simulink model "rx2"  (R2022b)
settings: Solver=FixedStepDiscrete  StartTime=0.0  StopTime=3.3E6  FixedStep=1  RelTol=1e-3  EnableMultiTasking=on
model workspace (MAT data in the model file):
  mwTaskManagerKernelLatency = 0
undefined symbols (not defined in the file or in its folder): Add, jsin, magnitude, rom_pilot_conj_tt, Shift
libraries: hdlsllib x3231, whdlutilities x525, simulink x260, whdlmod x112, whdledac x26, dsphdlmathfun2 x24, commchan3 x1
(part 19 of 59)

== system rx2/process divide/transport_block8/Subsystem4/ctrl_gen ==
  data_in : Inport
  valid_in : Inport  Port=2
  Delay : Delay  DelayLength=1  InitialCondition=0
  Delay1 : Delay  DelayLength=1  InitialCondition=0
  Delay2 : Delay  DelayLength=1  InitialCondition=0
  Detect Fall Nonpositive : hdlsllib/Logic and Bit Operations/Detect Fall Nonpositive  vinit=0  OutDataTypeStr=boolean
  Detect Rise Positive : hdlsllib/Logic and Bit Operations/Detect Rise Positive  vinit=0  OutDataTypeStr=boolean
  Sample Control Bus Creator : whdlutilities/Sample Control Bus Creator
  data_out : Outport
  ctrl_out : Outport  Port=2
  wires:
  Detect Fall Nonpositive/1 -> Sample Control Bus Creator/2
  valid_in/1 -> Delay/1, Detect Fall Nonpositive/1, Delay1/1
  Sample Control Bus Creator/1 -> ctrl_out/1
  Delay/1 -> Sample Control Bus Creator/3
  Delay1/1 -> Detect Rise Positive/1
  data_in/1 -> Delay2/1
  Delay2/1 -> data_out/1
  Detect Rise Positive/1 -> Sample Control Bus Creator/1

== system rx2/process divide/transport_block8/Subsystem5/ctrl_gen ==
  data_in : Inport
  valid_in : Inport  Port=2
  Delay : Delay  DelayLength=1  InitialCondition=0
  Delay1 : Delay  DelayLength=1  InitialCondition=0
  Delay2 : Delay  DelayLength=1  InitialCondition=0
  Detect Fall Nonpositive : hdlsllib/Logic and Bit Operations/Detect Fall Nonpositive  vinit=0  OutDataTypeStr=boolean
  Detect Rise Positive : hdlsllib/Logic and Bit Operations/Detect Rise Positive  vinit=0  OutDataTypeStr=boolean
  Sample Control Bus Creator : whdlutilities/Sample Control Bus Creator
  data_out : Outport
  ctrl_out : Outport  Port=2
  wires:
  Detect Fall Nonpositive/1 -> Sample Control Bus Creator/2
  valid_in/1 -> Delay/1, Detect Fall Nonpositive/1, Delay1/1
  Sample Control Bus Creator/1 -> ctrl_out/1
  Delay/1 -> Sample Control Bus Creator/3
  Delay1/1 -> Detect Rise Positive/1
  data_in/1 -> Delay2/1
  Delay2/1 -> data_out/1
  Detect Rise Positive/1 -> Sample Control Bus Creator/1

== system rx2/process divide/transport_block8/Subsystem6/ctrl_gen ==
  data_in : Inport
  valid_in : Inport  Port=2
  Delay : Delay  DelayLength=1  InitialCondition=0
  Delay1 : Delay  DelayLength=1  InitialCondition=0
  Delay2 : Delay  DelayLength=1  InitialCondition=0
  Detect Fall Nonpositive : hdlsllib/Logic and Bit Operations/Detect Fall Nonpositive  vinit=0  OutDataTypeStr=boolean
  Detect Rise Positive : hdlsllib/Logic and Bit Operations/Detect Rise Positive  vinit=0  OutDataTypeStr=boolean
  Sample Control Bus Creator : whdlutilities/Sample Control Bus Creator
  data_out : Outport
  ctrl_out : Outport  Port=2
  wires:
  Detect Fall Nonpositive/1 -> Sample Control Bus Creator/2
  valid_in/1 -> Delay/1, Detect Fall Nonpositive/1, Delay1/1
  Sample Control Bus Creator/1 -> ctrl_out/1
  Delay/1 -> Sample Control Bus Creator/3
  Delay1/1 -> Detect Rise Positive/1
  data_in/1 -> Delay2/1
  Delay2/1 -> data_out/1
  Detect Rise Positive/1 -> Sample Control Bus Creator/1

== system rx2/process divide/transport_block8/Subsystem7/ctrl_gen ==
  data_in : Inport
  valid_in : Inport  Port=2
  Delay : Delay  DelayLength=1  InitialCondition=0
  Delay1 : Delay  DelayLength=1  InitialCondition=0
  Delay2 : Delay  DelayLength=1  InitialCondition=0
  Detect Fall Nonpositive : hdlsllib/Logic and Bit Operations/Detect Fall Nonpositive  vinit=0  OutDataTypeStr=boolean
  Detect Rise Positive : hdlsllib/Logic and Bit Operations/Detect Rise Positive  vinit=0  OutDataTypeStr=boolean
  Sample Control Bus Creator : whdlutilities/Sample Control Bus Creator
  data_out : Outport
  ctrl_out : Outport  Port=2
  wires:
  Detect Fall Nonpositive/1 -> Sample Control Bus Creator/2
  valid_in/1 -> Delay/1, Detect Fall Nonpositive/1, Delay1/1
  Sample Control Bus Creator/1 -> ctrl_out/1
  Delay/1 -> Sample Control Bus Creator/3
  Delay1/1 -> Detect Rise Positive/1
  data_in/1 -> Delay2/1
  Delay2/1 -> data_out/1
  Detect Rise Positive/1 -> Sample Control Bus Creator/1

== system rx2/process divide/transport_block8/Subsystem8/ctrl_gen ==
  data_in : Inport
  valid_in : Inport  Port=2
  Delay : Delay  DelayLength=1  InitialCondition=0
  Delay1 : Delay  DelayLength=1  InitialCondition=0
  Delay2 : Delay  DelayLength=1  InitialCondition=0
  Detect Fall Nonpositive : hdlsllib/Logic and Bit Operations/Detect Fall Nonpositive  vinit=0  OutDataTypeStr=boolean
  Detect Rise Positive : hdlsllib/Logic and Bit Operations/Detect Rise Positive  vinit=0  OutDataTypeStr=boolean
  Sample Control Bus Creator : whdlutilities/Sample Control Bus Creator
  data_out : Outport
  ctrl_out : Outport  Port=2
  wires:
  Detect Fall Nonpositive/1 -> Sample Control Bus Creator/2
  valid_in/1 -> Delay/1, Detect Fall Nonpositive/1, Delay1/1
  Sample Control Bus Creator/1 -> ctrl_out/1
  Delay/1 -> Sample Control Bus Creator/3
  Delay1/1 -> Detect Rise Positive/1
  data_in/1 -> Delay2/1
  Delay2/1 -> data_out/1
  Detect Rise Positive/1 -> Sample Control Bus Creator/1

== system rx2/process divide/transport_block8/Subsystem9/ctrl_gen ==
  data_in : Inport
  valid_in : Inport  Port=2
  Delay : Delay  DelayLength=1  InitialCondition=0
  Delay1 : Delay  DelayLength=1  InitialCondition=0
  Delay2 : Delay  DelayLength=1  InitialCondition=0
  Detect Fall Nonpositive : hdlsllib/Logic and Bit Operations/Detect Fall Nonpositive  vinit=0  OutDataTypeStr=boolean
  Detect Rise Positive : hdlsllib/Logic and Bit Operations/Detect Rise Positive  vinit=0  OutDataTypeStr=boolean
  Sample Control Bus Creator : whdlutilities/Sample Control Bus Creator
  data_out : Outport
  ctrl_out : Outport  Port=2
  wires:
  Detect Fall Nonpositive/1 -> Sample Control Bus Creator/2
  valid_in/1 -> Delay/1, Detect Fall Nonpositive/1, Delay1/1
  Sample Control Bus Creator/1 -> ctrl_out/1
  Delay/1 -> Sample Control Bus Creator/3
  Delay1/1 -> Detect Rise Positive/1
  data_in/1 -> Delay2/1
  Delay2/1 -> data_out/1
  Detect Rise Positive/1 -> Sample Control Bus Creator/1

== system rx2/process1/OFDM_DEMOD1/OFDM_demod1/ctrl_gen ==
  data_in : Inport
  valid_in : Inport  Port=2
  Data Type Conversion : DataTypeConversion  OutDataTypeStr=fixdt(1,16,12)  SaturateOnIntegerOverflow=off  RndMeth=Floor
  Delay : Delay  DelayLength=1  InitialCondition=0
  Delay1 : Delay  DelayLength=1  InitialCondition=0
  Delay2 : Delay  DelayLength=1  InitialCondition=0
  Detect Fall Nonpositive : hdlsllib/Logic and Bit Operations/Detect Fall Nonpositive  vinit=0  OutDataTypeStr=boolean
  Detect Rise Positive : hdlsllib/Logic and Bit Operations/Detect Rise Positive  vinit=0  OutDataTypeStr=boolean
  Sample Control Bus Creator : whdlutilities/Sample Control Bus Creator
  data_out : Outport  OutDataTypeStr=fixdt(1,16,12)
  ctrl_out : Outport  Port=2
  wires:
  Detect Fall Nonpositive/1 -> Sample Control Bus Creator/2
  valid_in/1 -> Delay/1, Detect Fall Nonpositive/1, Delay1/1
  Sample Control Bus Creator/1 -> ctrl_out/1
  Delay/1 -> Sample Control Bus Creator/3
  Delay1/1 -> Detect Rise Positive/1
  data_in/1 -> Delay2/1
  Delay2/1 -> Data Type Conversion/1
  Detect Rise Positive/1 -> Sample Control Bus Creator/1
  Data Type Conversion/1 -> data_out/1

== system rx2/process1/OFDM_DEMOD1/OFDM_demod2/ctrl_gen ==
  data_in : Inport
  valid_in : Inport  Port=2
  Data Type Conversion : DataTypeConversion  OutDataTypeStr=fixdt(1,16,12)  SaturateOnIntegerOverflow=off  RndMeth=Floor
  Delay : Delay  DelayLength=1  InitialCondition=0
  Delay1 : Delay  DelayLength=1  InitialCondition=0
  Delay2 : Delay  DelayLength=1  InitialCondition=0
  Detect Fall Nonpositive : hdlsllib/Logic and Bit Operations/Detect Fall Nonpositive  vinit=0  OutDataTypeStr=boolean
  Detect Rise Positive : hdlsllib/Logic and Bit Operations/Detect Rise Positive  vinit=0  OutDataTypeStr=boolean
  Sample Control Bus Creator : whdlutilities/Sample Control Bus Creator
  data_out : Outport  OutDataTypeStr=fixdt(1,16,12)
  ctrl_out : Outport  Port=2
  wires:
  Detect Fall Nonpositive/1 -> Sample Control Bus Creator/2
  valid_in/1 -> Delay/1, Detect Fall Nonpositive/1, Delay1/1
  Sample Control Bus Creator/1 -> ctrl_out/1
  Delay/1 -> Sample Control Bus Creator/3
  Delay1/1 -> Detect Rise Positive/1
  data_in/1 -> Delay2/1
  Delay2/1 -> Data Type Conversion/1
  Detect Rise Positive/1 -> Sample Control Bus Creator/1
  Data Type Conversion/1 -> data_out/1

== system rx2/process1/OFDM_DEMOD1/OFDM_demod3/ctrl_gen ==
  data_in : Inport
  valid_in : Inport  Port=2
  Data Type Conversion : DataTypeConversion  OutDataTypeStr=fixdt(1,16,12)  SaturateOnIntegerOverflow=off  RndMeth=Floor
  Delay : Delay  DelayLength=1  InitialCondition=0
  Delay1 : Delay  DelayLength=1  InitialCondition=0
  Delay2 : Delay  DelayLength=1  InitialCondition=0
  Detect Fall Nonpositive : hdlsllib/Logic and Bit Operations/Detect Fall Nonpositive  vinit=0  OutDataTypeStr=boolean
  Detect Rise Positive : hdlsllib/Logic and Bit Operations/Detect Rise Positive  vinit=0  OutDataTypeStr=boolean
  Sample Control Bus Creator : whdlutilities/Sample Control Bus Creator
  data_out : Outport  OutDataTypeStr=fixdt(1,16,12)
  ctrl_out : Outport  Port=2
  wires:
  Detect Fall Nonpositive/1 -> Sample Control Bus Creator/2
  valid_in/1 -> Delay/1, Detect Fall Nonpositive/1, Delay1/1
  Sample Control Bus Creator/1 -> ctrl_out/1
  Delay/1 -> Sample Control Bus Creator/3
  Delay1/1 -> Detect Rise Positive/1
  data_in/1 -> Delay2/1
  Delay2/1 -> Data Type Conversion/1
  Detect Rise Positive/1 -> Sample Control Bus Creator/1
  Data Type Conversion/1 -> data_out/1

== system rx2/process1/OFDM_DEMOD1/OFDM_demod4/ctrl_gen ==
  data_in : Inport
  valid_in : Inport  Port=2
  Data Type Conversion : DataTypeConversion  OutDataTypeStr=fixdt(1,16,12)  SaturateOnIntegerOverflow=off  RndMeth=Floor
  Delay : Delay  DelayLength=1  InitialCondition=0
  Delay1 : Delay  DelayLength=1  InitialCondition=0
  Delay2 : Delay  DelayLength=1  InitialCondition=0
  Detect Fall Nonpositive : hdlsllib/Logic and Bit Operations/Detect Fall Nonpositive  vinit=0  OutDataTypeStr=boolean
  Detect Rise Positive : hdlsllib/Logic and Bit Operations/Detect Rise Positive  vinit=0  OutDataTypeStr=boolean
  Sample Control Bus Creator : whdlutilities/Sample Control Bus Creator
  data_out : Outport  OutDataTypeStr=fixdt(1,16,12)
  ctrl_out : Outport  Port=2
  wires:
  Detect Fall Nonpositive/1 -> Sample Control Bus Creator/2
  valid_in/1 -> Delay/1, Detect Fall Nonpositive/1, Delay1/1
  Sample Control Bus Creator/1 -> ctrl_out/1
  Delay/1 -> Sample Control Bus Creator/3
  Delay1/1 -> Detect Rise Positive/1
  data_in/1 -> Delay2/1
  Delay2/1 -> Data Type Conversion/1
  Detect Rise Positive/1 -> Sample Control Bus Creator/1
  Data Type Conversion/1 -> data_out/1

== system rx2/process1/OFDM_DEMOD1/OFDM_demod5/ctrl_gen ==
  data_in : Inport
  valid_in : Inport  Port=2
  Data Type Conversion : DataTypeConversion  OutDataTypeStr=fixdt(1,16,12)  SaturateOnIntegerOverflow=off  RndMeth=Floor
  Delay : Delay  DelayLength=1  InitialCondition=0
  Delay1 : Delay  DelayLength=1  InitialCondition=0
  Delay2 : Delay  DelayLength=1  InitialCondition=0
  Detect Fall Nonpositive : hdlsllib/Logic and Bit Operations/Detect Fall Nonpositive  vinit=0  OutDataTypeStr=boolean
  Detect Rise Positive : hdlsllib/Logic and Bit Operations/Detect Rise Positive  vinit=0  OutDataTypeStr=boolean
  Sample Control Bus Creator : whdlutilities/Sample Control Bus Creator
  data_out : Outport  OutDataTypeStr=fixdt(1,16,12)
  ctrl_out : Outport  Port=2
  wires:
  Detect Fall Nonpositive/1 -> Sample Control Bus Creator/2
  valid_in/1 -> Delay/1, Detect Fall Nonpositive/1, Delay1/1
  Sample Control Bus Creator/1 -> ctrl_out/1
  Delay/1 -> Sample Control Bus Creator/3
  Delay1/1 -> Detect Rise Positive/1
  data_in/1 -> Delay2/1
  Delay2/1 -> Data Type Conversion/1
  Detect Rise Positive/1 -> Sample Control Bus Creator/1
  Data Type Conversion/1 -> data_out/1

== system rx2/process1/OFDM_DEMOD1/OFDM_demod6/ctrl_gen ==
  data_in : Inport
  valid_in : Inport  Port=2
  Data Type Conversion : DataTypeConversion  OutDataTypeStr=fixdt(1,16,12)  SaturateOnIntegerOverflow=off  RndMeth=Floor
  Delay : Delay  DelayLength=1  InitialCondition=0
  Delay1 : Delay  DelayLength=1  InitialCondition=0
  Delay2 : Delay  DelayLength=1  InitialCondition=0
  Detect Fall Nonpositive : hdlsllib/Logic and Bit Operations/Detect Fall Nonpositive  vinit=0  OutDataTypeStr=boolean
  Detect Rise Positive : hdlsllib/Logic and Bit Operations/Detect Rise Positive  vinit=0  OutDataTypeStr=boolean
  Sample Control Bus Creator : whdlutilities/Sample Control Bus Creator
  data_out : Outport  OutDataTypeStr=fixdt(1,16,12)
  ctrl_out : Outport  Port=2
  wires:
  Detect Fall Nonpositive/1 -> Sample Control Bus Creator/2
  valid_in/1 -> Delay/1, Detect Fall Nonpositive/1, Delay1/1
  Sample Control Bus Creator/1 -> ctrl_out/1
  Delay/1 -> Sample Control Bus Creator/3
  Delay1/1 -> Detect Rise Positive/1
  data_in/1 -> Delay2/1
  Delay2/1 -> Data Type Conversion/1
  Detect Rise Positive/1 -> Sample Control Bus Creator/1
  Data Type Conversion/1 -> data_out/1

== system rx2/process1/OFDM_DEMOD1/OFDM_demod7/ctrl_gen ==
  data_in : Inport
  valid_in : Inport  Port=2
  Data Type Conversion : DataTypeConversion  OutDataTypeStr=fixdt(1,16,12)  SaturateOnIntegerOverflow=off  RndMeth=Floor
  Delay : Delay  DelayLength=1  InitialCondition=0
  Delay1 : Delay  DelayLength=1  InitialCondition=0
  Delay2 : Delay  DelayLength=1  InitialCondition=0
  Detect Fall Nonpositive : hdlsllib/Logic and Bit Operations/Detect Fall Nonpositive  vinit=0  OutDataTypeStr=boolean
  Detect Rise Positive : hdlsllib/Logic and Bit Operations/Detect Rise Positive  vinit=0  OutDataTypeStr=boolean
  Sample Control Bus Creator : whdlutilities/Sample Control Bus Creator
  data_out : Outport  OutDataTypeStr=fixdt(1,16,12)
  ctrl_out : Outport  Port=2
  wires:
  Detect Fall Nonpositive/1 -> Sample Control Bus Creator/2
  valid_in/1 -> Delay/1, Detect Fall Nonpositive/1, Delay1/1
  Sample Control Bus Creator/1 -> ctrl_out/1
  Delay/1 -> Sample Control Bus Creator/3
  Delay1/1 -> Detect Rise Positive/1
  data_in/1 -> Delay2/1
  Delay2/1 -> Data Type Conversion/1
  Detect Rise Positive/1 -> Sample Control Bus Creator/1
  Data Type Conversion/1 -> data_out/1

== system rx2/process1/OFDM_DEMOD1/OFDM_demod8/ctrl_gen ==
  data_in : Inport
  valid_in : Inport  Port=2
  Data Type Conversion : DataTypeConversion  OutDataTypeStr=fixdt(1,16,12)  SaturateOnIntegerOverflow=off  RndMeth=Floor
  Delay : Delay  DelayLength=1  InitialCondition=0
  Delay1 : Delay  DelayLength=1  InitialCondition=0
  Delay2 : Delay  DelayLength=1  InitialCondition=0
  Detect Fall Nonpositive : hdlsllib/Logic and Bit Operations/Detect Fall Nonpositive  vinit=0  OutDataTypeStr=boolean
  Detect Rise Positive : hdlsllib/Logic and Bit Operations/Detect Rise Positive  vinit=0  OutDataTypeStr=boolean
  Sample Control Bus Creator : whdlutilities/Sample Control Bus Creator
  data_out : Outport  OutDataTypeStr=fixdt(1,16,12)
  ctrl_out : Outport  Port=2
  wires:
  Detect Fall Nonpositive/1 -> Sample Control Bus Creator/2
  valid_in/1 -> Delay/1, Detect Fall Nonpositive/1, Delay1/1
  Sample Control Bus Creator/1 -> ctrl_out/1
  Delay/1 -> Sample Control Bus Creator/3
  Delay1/1 -> Detect Rise Positive/1
  data_in/1 -> Delay2/1
  Delay2/1 -> Data Type Conversion/1
  Detect Rise Positive/1 -> Sample Control Bus Creator/1
  Data Type Conversion/1 -> data_out/1

== system rx2/process1/decoder/deinterleave/Subsystem ==
  start : Inport
  Compare To Constant : simulink/Logic and Bit Operations/Compare To Constant  relop===  const=valid_length  OutDataTypeStr=boolean
  Data Type Conversion : DataTypeConversion  OutDataTypeStr=boolean  SaturateOnIntegerOverflow=off  RndMeth=Floor
  Delay2 : Delay  DelayLength=1  InitialCondition=0
  HDL Counter1 : hdlsllib/Sources/HDL Counter  CountType=Count limited  CountInit=1  CountStep=1  CountMax=valid_length  CountFromType=Initial value  CountFrom=1  CountResetPort=off  CountLoadPort=off  CountEnbPort=on  CountDirPort=off  CountHitOutputPort=off  CountDataType=Unsigned  CountWordLen=16  CountFracLen=0  CountSampTime=1
  HDL Counter4 : hdlsllib/Sources/HDL Counter  CountType=Count limited  CountInit=0  CountStep=1  CountMax=1  CountFromType=Initial value  CountFrom=0  CountResetPort=on  CountLoadPort=off  CountEnbPort=on  CountDirPort=off  CountHitOutputPort=off  CountDataType=Unsigned  CountWordLen=8  CountFracLen=0  CountSampTime=1
  valid_out : Outport
  wires:
  Compare To Constant/1 -> HDL Counter4/1
  HDL Counter1/1 -> Compare To Constant/1  "count_1"
  HDL Counter4/1 -> Data Type Conversion/1
  start/1 -> HDL Counter4/2
  Data Type Conversion/1 -> Delay2/1, HDL Counter1/1
  Delay2/1 -> valid_out/1  "valid_out"

== system rx2/process1/decoder/deinterleave/Subsystem1 ==
  start : Inport
  Compare To Constant : simulink/Logic and Bit Operations/Compare To Constant  relop===  const=valid_length  OutDataTypeStr=boolean
  Data Type Conversion : DataTypeConversion  OutDataTypeStr=boolean  SaturateOnIntegerOverflow=off  RndMeth=Floor
  Delay2 : Delay  DelayLength=1  InitialCondition=0
  HDL Counter1 : hdlsllib/Sources/HDL Counter  CountType=Count limited  CountInit=1  CountStep=1  CountMax=valid_length  CountFromType=Initial value  CountFrom=1  CountResetPort=off  CountLoadPort=off  CountEnbPort=on  CountDirPort=off  CountHitOutputPort=off  CountDataType=Unsigned  CountWordLen=16  CountFracLen=0  CountSampTime=1
  HDL Counter4 : hdlsllib/Sources/HDL Counter  CountType=Count limited  CountInit=0  CountStep=1  CountMax=1  CountFromType=Initial value  CountFrom=0  CountResetPort=on  CountLoadPort=off  CountEnbPort=on  CountDirPort=off  CountHitOutputPort=off  CountDataType=Unsigned  CountWordLen=8  CountFracLen=0  CountSampTime=1
  valid_out : Outport
  wires:
  Compare To Constant/1 -> HDL Counter4/1
  HDL Counter1/1 -> Compare To Constant/1  "count_1"
  HDL Counter4/1 -> Data Type Conversion/1
  start/1 -> HDL Counter4/2
  Data Type Conversion/1 -> Delay2/1, HDL Counter1/1
  Delay2/1 -> valid_out/1  "valid_out"

== system rx2/process1/decoder/p-p/Subsystem ==
  start : Inport
  Compare To Constant : simulink/Logic and Bit Operations/Compare To Constant  relop===  const=valid_length  OutDataTypeStr=boolean
  Data Type Conversion : DataTypeConversion  OutDataTypeStr=boolean  SaturateOnIntegerOverflow=off  RndMeth=Floor
  Delay1 : Delay  InitialCondition=0
  Delay2 : Delay  DelayLength=1  InitialCondition=0
  Detect Fall Nonpositive : simulink/Logic and Bit Operations/Detect Fall Nonpositive  vinit=0  OutDataTypeStr=boolean
  HDL Counter1 : hdlsllib/Sources/HDL Counter  CountType=Count limited  CountInit=1  CountStep=1  CountMax=valid_length  CountFromType=Initial value  CountFrom=1  CountResetPort=off  CountLoadPort=off  CountEnbPort=on  CountDirPort=off  CountHitOutputPort=off  CountDataType=Unsigned  CountWordLen=16  CountFracLen=0  CountSampTime=1
  HDL Counter4 : hdlsllib/Sources/HDL Counter  CountType=Count limited  CountInit=0  CountStep=1  CountMax=1  CountFromType=Initial value  CountFrom=0  CountResetPort=on  CountLoadPort=off  CountEnbPort=on  CountDirPort=off  CountHitOutputPort=off  CountDataType=Unsigned  CountWordLen=8  CountFracLen=0  CountSampTime=1
  Logical Operator4 : Logic  AllPortsSameDT=off  OutDataTypeStr=boolean
  valid_out : Outport
  start_out : Outport  Port=2
  end_out : Outport  Port=3
  wires:
  Compare To Constant/1 -> HDL Counter4/1
  HDL Counter1/1 -> Compare To Constant/1  "count_1"
  HDL Counter4/1 -> Data Type Conversion/1
  start/1 -> Delay1/1, HDL Counter4/2
  Detect Fall Nonpositive/1 -> Logical Operator4/1  "symbol_end"
  Data Type Conversion/1 -> Delay2/1, Detect Fall Nonpositive/1, HDL Counter1/1
  Delay1/1 -> start_out/1  "start_out"
  Delay2/1 -> Logical Operator4/2, valid_out/1  "valid_out"
  Logical Operator4/1 -> end_out/1  "end_out"

== system rx2/process1/decoder/p-p/Subsystem2 ==
  data1 : Inport  OutDataTypeStr=data_type
  wr_addr : Inport  Port=2
  wr_en1 : Inport  Port=3
  rd_addr : Inport  Port=4
  Mux : Mux  Inputs=2
  Selector : Selector  InputPortWidth=64  IndexOptions=Index vector (dialog)  Indices=[1:32]  OutputSizes=1
  Selector1 : Selector  InputPortWidth=64  IndexOptions=Index vector (dialog)  Indices=[33:64]  OutputSizes=1
  Subsystem : Subsystem
  Subsystem1 : Subsystem
  rd_dout : Outport  PortDimensions=64  VectorParamsAs1DForOutWhenUnconnected=off
  wires:
  rd_addr/1 -> Subsystem1/4(rd_addr), Subsystem/4(rd_addr)
  data1/1 -> Selector1/1, Selector/1
  Subsystem/1(rd_dout) -> Mux/1
  Subsystem1/1(rd_dout) -> Mux/2
  Selector1/1 -> Subsystem1/1(data1)
  Selector/1 -> Subsystem/1(data1)
  wr_en1/1 -> Subsystem1/3(wr_en1), Subsystem/3(wr_en1)
  wr_addr/1 -> Subsystem1/2(wr_addr), Subsystem/2(wr_addr)
  Mux/1 -> rd_dout/1

== system rx2/process1/decoder/p-p/p_s_new ==
  data_in : Inport
  valid : Inport  Port=2
  end : Inport  Port=3
  Demux{,1..34} (35 alike) : Demux  Outputs=2
  Ground : Ground
  HDL Counter3 : hdlsllib/Sources/HDL Counter  CountType=Count limited  CountInit=1  CountStep=1  CountMax=64  CountFromType=Specify  CountFrom=1  CountResetPort=on  CountLoadPort=off  CountEnbPort=on  CountDirPort=off  CountHitOutputPort=off  CountDataType=Unsigned  CountWordLen=16  CountFracLen=0  CountSampTime=1
  Multiport Switch : MultiPortSwitch  Inputs=64  DataPortForDefault=Additional data port  DiagnosticForDefault=None  SaturateOnIntegerOverflow=off  InputSameDT=off
  Subsystem1 : Subsystem
  Subsystem3 : Subsystem
  Subsystem4 : Subsystem
  Subsystem5 : Subsystem
  data_out : Outport
  wires:
  Subsystem4/4(Out4) -> Demux17/1
  Demux14/2 -> Multiport Switch/49
  Subsystem1/2(Out2) -> Demux2/1
  Demux24/2 -> Multiport Switch/55
  Demux6/1 -> Multiport Switch/8
  Demux22/1 -> Multiport Switch/64
  Demux/1 -> Demux3/1
  Demux18/1 -> Multiport Switch/42
  Subsystem4/1(Out1) -> Demux13/1
  Subsystem4/3(Out3) -> Demux16/1
  Demux27/2 -> Multiport Switch/61
  Demux4/2 -> Subsystem5/1(In1)
  Demux13/2 -> Multiport Switch/35
  Demux5/1 -> Multiport Switch/6
  Demux9/1 -> Multiport Switch/14
  Subsystem4/2(Out2) -> Demux15/1
  Demux8/2 -> Multiport Switch/13
  Demux20/2 -> Multiport Switch/47
  Subsystem4/8(Out8) -> Demux14/1
  Subsystem5/4(Out4) -> Demux25/1
  Subsystem4/6(Out6) -> Demux19/1
  Subsystem4/5(Out5) -> Demux18/1
  Demux7/2 -> Multiport Switch/11
  Subsystem4/7(Out7) -> Demux20/1
  Demux14/1 -> Multiport Switch/48
  Demux19/1 -> Multiport Switch/44
  Demux20/1 -> Multiport Switch/46
  Subsystem5/2(Out2) -> Demux23/1
  Demux5/2 -> Multiport Switch/7
  Demux16/1 -> Multiport Switch/38
  Demux17/1 -> Multiport Switch/40
  Subsystem5/8(Out8) -> Demux22/1
  Demux22/2 -> Multiport Switch/65
  Demux13/1 -> Multiport Switch/34
  Demux21/2 -> Multiport Switch/51
  Demux16/2 -> Multiport Switch/39
  Demux3/2 -> Subsystem3/1(In1)
  Demux19/2 -> Multiport Switch/45
  Demux15/2 -> Multiport Switch/37
  Demux26/1 -> Multiport Switch/58
  Demux25/2 -> Multiport Switch/57
  Subsystem3/6(Out6) -> Demux33/1
  Subsystem3/7(Out7) -> Demux34/1
  Demux18/2 -> Multiport Switch/43
  Demux23/2 -> Multiport Switch/53
  Demux1/2 -> Multiport Switch/3
  Subsystem3/8(Out8) -> Demux12/1
  Demux17/2 -> Multiport Switch/41
  Subsystem5/3(Out3) -> Demux24/1
  Subsystem1/3(Out3) -> Demux5/1
  Demux23/1 -> Multiport Switch/52
  Subsystem1/5(Out5) -> Demux7/1
  Demux24/1 -> Multiport Switch/54
  Demux32/1 -> Multiport Switch/26
  Subsystem3/5(Out5) -> Demux32/1
  Demux21/1 -> Multiport Switch/50
  Demux25/1 -> Multiport Switch/56
  Demux28/2 -> Multiport Switch/63
  Demux26/2 -> Multiport Switch/59
  Demux27/1 -> Multiport Switch/60
  Subsystem5/6(Out6) -> Demux27/1
  Demux28/1 -> Multiport Switch/62
  Subsystem1/1(Out1) -> Demux1/1
  Demux4/1 -> Subsystem4/1(In1)
  Demux2/2 -> Multiport Switch/5
  Subsystem1/7(Out7) -> Demux9/1
  Demux15/1 -> Multiport Switch/36
  Subsystem5/7(Out7) -> Demux28/1
  Subsystem5/5(Out5) -> Demux26/1
  Demux29/1 -> Multiport Switch/20
  Subsystem5/1(Out1) -> Demux21/1
  Subsystem1/6(Out6) -> Demux8/1
  Demux8/1 -> Multiport Switch/12
  Demux1/1 -> Multiport Switch/2
  Subsystem1/8(Out8) -> Demux10/1
  Demux10/2 -> Multiport Switch/17
  Demux10/1 -> Multiport Switch/16
  Demux32/2 -> Multiport Switch/27
  Demux2/1 -> Multiport Switch/4
  Demux6/2 -> Multiport Switch/9
  Demux34/1 -> Multiport Switch/30
  Subsystem3/1(Out1) -> Demux11/1
  Subsystem3/4(Out4) -> Demux31/1
  Subsystem3/2(Out2) -> Demux29/1
  Subsystem3/3(Out3) -> Demux30/1
  Demux3/1 -> Subsystem1/1(In1)
  Demux29/2 -> Multiport Switch/21
  Demux33/1 -> Multiport Switch/28
  Demux30/1 -> Multiport Switch/22
  Demux34/2 -> Multiport Switch/31
  Demux11/1 -> Multiport Switch/18
  Demux12/1 -> Multiport Switch/32
  Demux11/2 -> Multiport Switch/19
  Demux12/2 -> Multiport Switch/33
  Demux31/1 -> Multiport Switch/24
  Demux33/2 -> Multiport Switch/29
  Demux30/2 -> Multiport Switch/23
  Demux31/2 -> Multiport Switch/25
  Subsystem1/4(Out4) -> Demux6/1
  Demux/2 -> Demux4/1
  Demux9/2 -> Multiport Switch/15
  Demux7/1 -> Multiport Switch/10
  valid/1 -> HDL Counter3/2
  Multiport Switch/1 -> data_out/1
  data_in/1 -> Demux/1
  HDL Counter3/1 -> Multiport Switch/1
  end/1 -> HDL Counter3/1
  Ground/1 -> Multiport Switch/66

== system rx2/process1/decoder/rate recover/Subsystem ==
  start : Inport
  Compare To Constant : simulink/Logic and Bit Operations/Compare To Constant  relop===  const=valid_length  OutDataTypeStr=boolean
  Data Type Conversion : DataTypeConversion  OutDataTypeStr=boolean  SaturateOnIntegerOverflow=off  RndMeth=Floor
  Delay1 : Delay  InitialCondition=0
  Delay2 : Delay  DelayLength=1  InitialCondition=0
  Detect Fall Nonpositive : simulink/Logic and Bit Operations/Detect Fall Nonpositive  vinit=0  OutDataTypeStr=boolean
  HDL Counter1 : hdlsllib/Sources/HDL Counter  CountType=Count limited  CountInit=1  CountStep=1  CountMax=valid_length  CountFromType=Initial value  CountFrom=1  CountResetPort=off  CountLoadPort=off  CountEnbPort=on  CountDirPort=off  CountHitOutputPort=off  CountDataType=Unsigned  CountWordLen=16  CountFracLen=0  CountSampTime=1
  HDL Counter4 : hdlsllib/Sources/HDL Counter  CountType=Count limited  CountInit=0  CountStep=1  CountMax=1  CountFromType=Initial value  CountFrom=0  CountResetPort=on  CountLoadPort=off  CountEnbPort=on  CountDirPort=off  CountHitOutputPort=off  CountDataType=Unsigned  CountWordLen=8  CountFracLen=0  CountSampTime=1
  Logical Operator4 : Logic  AllPortsSameDT=off  OutDataTypeStr=boolean
  valid_out : Outport
  start_out : Outport  Port=2
  end_out : Outport  Port=3
  wires:
  Compare To Constant/1 -> HDL Counter4/1
  HDL Counter1/1 -> Compare To Constant/1  "count_1"
  HDL Counter4/1 -> Data Type Conversion/1
  start/1 -> Delay1/1, HDL Counter4/2
  Detect Fall Nonpositive/1 -> Logical Operator4/1  "symbol_end"
  Data Type Conversion/1 -> Delay2/1, Detect Fall Nonpositive/1, HDL Counter1/1
  Delay1/1 -> start_out/1  "start_out"
  Delay2/1 -> Logical Operator4/2, valid_out/1  "valid_out"
  Logical Operator4/1 -> end_out/1  "end_out"

== system rx2/process1/decoder/s-p/S-P ==
  data_in : Inport  OutDataTypeStr=fixdt(1,16,9)
  valid_in : Inport  Port=2  OutDataTypeStr=boolean
  Deserializer1D : hdlsllib/HDL Operations/Deserializer1D  Ratio=data_len  IdleCycles=8  InitialCondition=0  startIn=off  validIn=on  validOut=on  inputDataDimensions=-1  inputSampleTime=1  inputSignalType=real
  Rate Transition : RateTransition  OutPortSampleTimeOpt=Multiple of input port sample time  OutPortSampleTimeMultiple=1/72
  Rate Transition1 : RateTransition  OutPortSampleTimeOpt=Multiple of input port sample time  OutPortSampleTimeMultiple=1/72
  data_out : Outport  OutDataTypeStr=fixdt(1,16,9)
  valid_out : Outport  Port=2  OutDataTypeStr=boolean
  wires:
  Deserializer1D/1 -> Rate Transition/1
  data_in/1 -> Deserializer1D/1
  Rate Transition/1 -> data_out/1  "data"
  Deserializer1D/2 -> Rate Transition1/1
  Rate Transition1/1 -> valid_out/1  "valid"
  valid_in/1 -> Deserializer1D/2  "valid_in"

== system rx2/process1/decoder/s-p/S-P2 ==
  data_in : Inport  OutDataTypeStr=fixdt(1,16,9)
  valid_in : Inport  Port=2  OutDataTypeStr=boolean
  Deserializer1D : hdlsllib/HDL Operations/Deserializer1D  Ratio=data_len  IdleCycles=64  InitialCondition=0  startIn=off  validIn=on  validOut=on  inputDataDimensions=-1  inputSampleTime=1  inputSignalType=real
  Rate Transition : RateTransition  OutPortSampleTimeOpt=Multiple of input port sample time  OutPortSampleTimeMultiple=1/72
  Rate Transition1 : RateTransition  OutPortSampleTimeOpt=Multiple of input port sample time  OutPortSampleTimeMultiple=1/72
  data_out : Outport  OutDataTypeStr=fixdt(1,16,9)
  valid_out : Outport  Port=2  OutDataTypeStr=boolean
  wires:
  Deserializer1D/1 -> Rate Transition/1
  data_in/1 -> Deserializer1D/1
  Rate Transition/1 -> data_out/1  "data"
  Deserializer1D/2 -> Rate Transition1/1
  Rate Transition1/1 -> valid_out/1  "valid"
  valid_in/1 -> Deserializer1D/2  "valid_in"

== system rx2/process1/decoder/soft demodule/Subsystem ==
  start : Inport
  Compare To Constant : simulink/Logic and Bit Operations/Compare To Constant  relop===  const=valid_length  OutDataTypeStr=boolean
  Data Type Conversion : DataTypeConversion  OutDataTypeStr=boolean  SaturateOnIntegerOverflow=off  RndMeth=Floor
  Delay1 : Delay  InitialCondition=0
  Delay2 : Delay  DelayLength=1  InitialCondition=0
  Detect Fall Nonpositive : simulink/Logic and Bit Operations/Detect Fall Nonpositive  vinit=0  OutDataTypeStr=boolean
  HDL Counter1 : hdlsllib/Sources/HDL Counter  CountType=Count limited  CountInit=1  CountStep=1  CountMax=valid_length  CountFromType=Initial value  CountFrom=1  CountResetPort=off  CountLoadPort=off  CountEnbPort=on  CountDirPort=off  CountHitOutputPort=off  CountDataType=Unsigned  CountWordLen=16  CountFracLen=0  CountSampTime=1
  HDL Counter4 : hdlsllib/Sources/HDL Counter  CountType=Count limited  CountInit=0  CountStep=1  CountMax=1  CountFromType=Initial value  CountFrom=0  CountResetPort=on  CountLoadPort=off  CountEnbPort=on  CountDirPort=off  CountHitOutputPort=off  CountDataType=Unsigned  CountWordLen=8  CountFracLen=0  CountSampTime=1
  Logical Operator4 : Logic  AllPortsSameDT=off  OutDataTypeStr=boolean
  valid_out : Outport
  start_out : Outport  Port=2
  end_out : Outport  Port=3
  wires:
  Compare To Constant/1 -> HDL Counter4/1
  HDL Counter1/1 -> Compare To Constant/1  "count_1"
  HDL Counter4/1 -> Data Type Conversion/1
  start/1 -> Delay1/1, HDL Counter4/2
  Detect Fall Nonpositive/1 -> Logical Operator4/1  "symbol_end"
  Data Type Conversion/1 -> Delay2/1, Detect Fall Nonpositive/1, HDL Counter1/1
  Delay1/1 -> start_out/1  "start_out"
  Delay2/1 -> Logical Operator4/2, valid_out/1  "valid_out"
  Logical Operator4/1 -> end_out/1  "end_out"

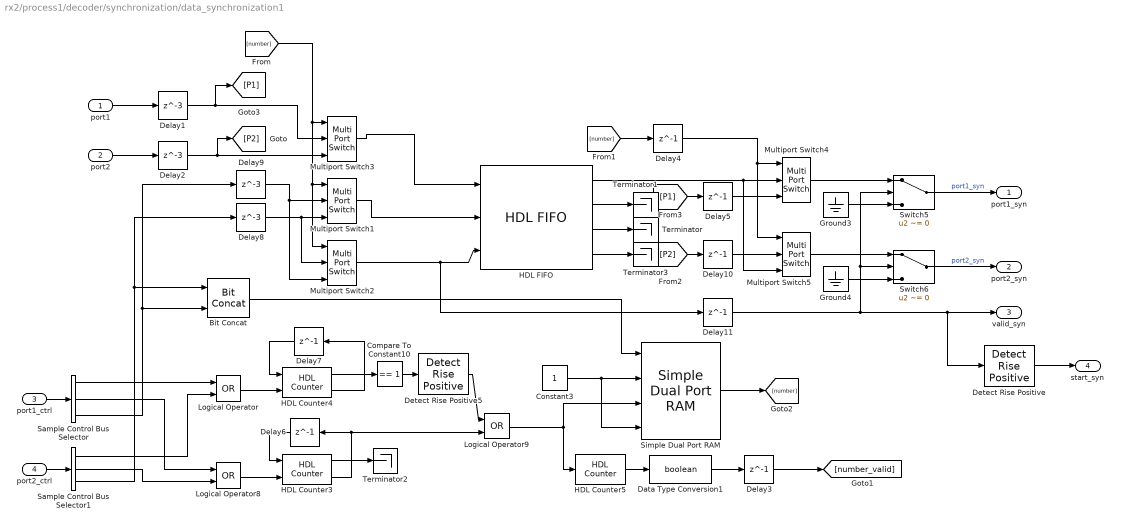
== system rx2/process1/decoder/synchronization/data_synchronization1 ==
  port1 : Inport
  port2 : Inport  Port=2
  port1_ctrl : Inport  Port=3  OutDataTypeStr=Bus: samplecontrol
  port2_ctrl : Inport  Port=4  OutDataTypeStr=Bus: samplecontrol
  Bit Concat : hdlsllib/Logic and Bit Operations/Bit Concat  numInputs=2
  Compare To Constant10 : hdlsllib/Logic and Bit Operations/Compare To Constant  relop===  const=1  OutDataTypeStr=boolean
  Constant3 : Constant  OutDataTypeStr=fixdt(0,2,0)
  Data Type Conversion1 : DataTypeConversion  OutDataTypeStr=boolean  SaturateOnIntegerOverflow=off  RndMeth=Floor
  Delay1 : Delay  DelayLength=3  InitialCondition=0  SampleTime=1
  Delay{3..7,10..11} (7 alike) : Delay  DelayLength=1  InitialCondition=0
  Delay2 : Delay  DelayLength=3  InitialCondition=0  SampleTime=1
  Delay8 : Delay  DelayLength=3  InitialCondition=0
  Delay9 : Delay  DelayLength=3  InitialCondition=0
  Detect Rise Positive : simulink/Logic and Bit Operations/Detect Rise Positive  vinit=0  OutDataTypeStr=boolean
  Detect Rise Positive5 : hdlsllib/Logic and Bit Operations/Detect Rise Positive  vinit=0  OutDataTypeStr=boolean
  Ground3 : Ground
  Ground4 : Ground
  HDL Counter3 : hdlsllib/Sources/HDL Counter  CountType=Count limited  CountInit=0  CountStep=1  CountMax=2  CountFromType=Initial value  CountFrom=0  CountResetPort=on  CountLoadPort=off  CountEnbPort=on  CountDirPort=off  CountHitOutputPort=on  CountDataType=Unsigned  CountWordLen=2  CountFracLen=0  CountSampTime=1
  HDL Counter4 : hdlsllib/Sources/HDL Counter  CountType=Count limited  CountInit=0  CountStep=1  CountMax=2  CountFromType=Initial value  CountFrom=0  CountResetPort=on  CountLoadPort=off  CountEnbPort=on  CountDirPort=off  CountHitOutputPort=on  CountDataType=Unsigned  CountWordLen=2  CountFracLen=0  CountSampTime=1
  HDL Counter5 : hdlsllib/Sources/HDL Counter  CountType=Count limited  CountInit=0  CountStep=1  CountMax=1  CountFromType=Initial value  CountFrom=0  CountResetPort=off  CountLoadPort=off  CountEnbPort=on  CountDirPort=off  CountHitOutputPort=off  CountDataType=Unsigned  CountWordLen=1  CountFracLen=0  CountSampTime=1
  HDL FIFO : hdlsllib/HDL RAMs/HDL FIFO  fifo_size=792  mode=Classic  ratio=1  push_msg=Warning  pop_msg=Ignore  show_empty=on  show_full=on  show_num=on  LabelModeActiveChoice_Mode=Classic  rst_port=off
  Logical Operator : Logic  Operator=OR  AllPortsSameDT=off  OutDataTypeStr=boolean
  Logical Operator8 : Logic  Operator=OR  AllPortsSameDT=off  OutDataTypeStr=boolean
  Logical Operator9 : Logic  Operator=OR  AllPortsSameDT=off  OutDataTypeStr=boolean
  Multiport Switch{1..5} (5 alike) : MultiPortSwitch  Inputs=2  DiagnosticForDefault=None  SaturateOnIntegerOverflow=off  InputSameDT=off
  Sample Control Bus Selector : whdlutilities/Sample Control Bus Selector  OutputSignals=start,end,valid
  Sample Control Bus Selector1 : whdlutilities/Sample Control Bus Selector  OutputSignals=start,end,valid
  Simple Dual Port RAM : hdlsllib/HDL RAMs/Simple Dual Port RAM  ram_size=2
  Switch5 : Switch  Criteria=u2 ~= 0  SaturateOnIntegerOverflow=off  InputSameDT=off
  Switch6 : Switch  Criteria=u2 ~= 0  SaturateOnIntegerOverflow=off  InputSameDT=off
  Terminator{,1..3} (4 alike) : Terminator
  port1_syn : Outport  VectorParamsAs1DForOutWhenUnconnected=off
  port2_syn : Outport  Port=2  VectorParamsAs1DForOutWhenUnconnected=off
  valid_syn : Outport  Port=3  OutDataTypeStr=boolean  VectorParamsAs1DForOutWhenUnconnected=off
  start_syn : Outport  Port=4  OutDataTypeStr=boolean  VectorParamsAs1DForOutWhenUnconnected=off
  wires:
  Detect Rise Positive/1 -> start_syn/1
  Delay11/1 -> valid_syn/1, Detect Rise Positive/1, Switch6/2, Switch5/2
  Multiport Switch5/1 -> Switch6/1
  Multiport Switch4/1 -> Switch5/1
  Ground3/1 -> Switch5/3
  Switch6/1 -> port2_syn/1  "port2_syn"
  Switch5/1 -> port1_syn/1  "port1_syn"
  Ground4/1 -> Switch6/3
  Delay5/1 -> Multiport Switch4/3
  Delay10/1 -> Multiport Switch5/2
  [P2] -> Delay10/1
  [P1] -> Delay5/1
  Delay1/1 -> Multiport Switch3/2, [P1]
  Delay4/1 -> Multiport Switch4/1, Multiport Switch5/1
  [number] -> Delay4/1
  HDL FIFO/4 -> Terminator3/1
  HDL FIFO/2 -> Terminator1/1
  Delay9/1 -> Multiport Switch1/2, Multiport Switch2/3
  Delay8/1 -> Multiport Switch1/3, Multiport Switch2/2
  Delay3/1 -> [number_valid]
  Delay2/1 -> Multiport Switch3/3, [P2]
  Sample Control Bus Selector1/3 -> Bit Concat/1, Delay8/1
  Sample Control Bus Selector/3 -> Bit Concat/2, Delay9/1
  [number] -> Multiport Switch3/1, Multiport Switch1/1, Multiport Switch2/1
  Multiport Switch2/1 -> HDL FIFO/3, Delay11/1
  Multiport Switch3/1 -> HDL FIFO/1
  HDL FIFO/3 -> Terminator/1
  HDL FIFO/1 -> Multiport Switch4/2, Multiport Switch5/3
  Multiport Switch1/1 -> HDL FIFO/2
  port2/1 -> Delay2/1
  port1/1 -> Delay1/1
  Simple Dual Port RAM/1 -> [number]
  Sample Control Bus Selector1/2 -> Logical Operator8/2
  Data Type Conversion1/1 -> Delay3/1
  Constant3/1 -> Simple Dual Port RAM/2, Simple Dual Port RAM/4
  Bit Concat/1 -> Simple Dual Port RAM/1
  Logical Operator9/1 -> Simple Dual Port RAM/3, HDL Counter5/1
  HDL Counter5/1 -> Data Type Conversion1/1
  HDL Counter4/1 -> Compare To Constant10/1
  Detect Rise Positive5/1 -> Logical Operator9/1
  Logical Operator/1 -> HDL Counter4/2
  Delay6/1 -> HDL Counter3/1
  HDL Counter3/1 -> Terminator2/1
  HDL Counter3/2 -> Delay6/1, Logical Operator9/2
  Logical Operator8/1 -> HDL Counter3/2
  Compare To Constant10/1 -> Detect Rise Positive5/1
  HDL Counter4/2 -> Delay7/1
  Delay7/1 -> HDL Counter4/1
  Sample Control Bus Selector/2 -> Logical Operator8/1
  Sample Control Bus Selector1/1 -> Logical Operator/2
  Sample Control Bus Selector/1 -> Logical Operator/1
  port2_ctrl/1 -> Sample Control Bus Selector1/1
  port1_ctrl/1 -> Sample Control Bus Selector/1

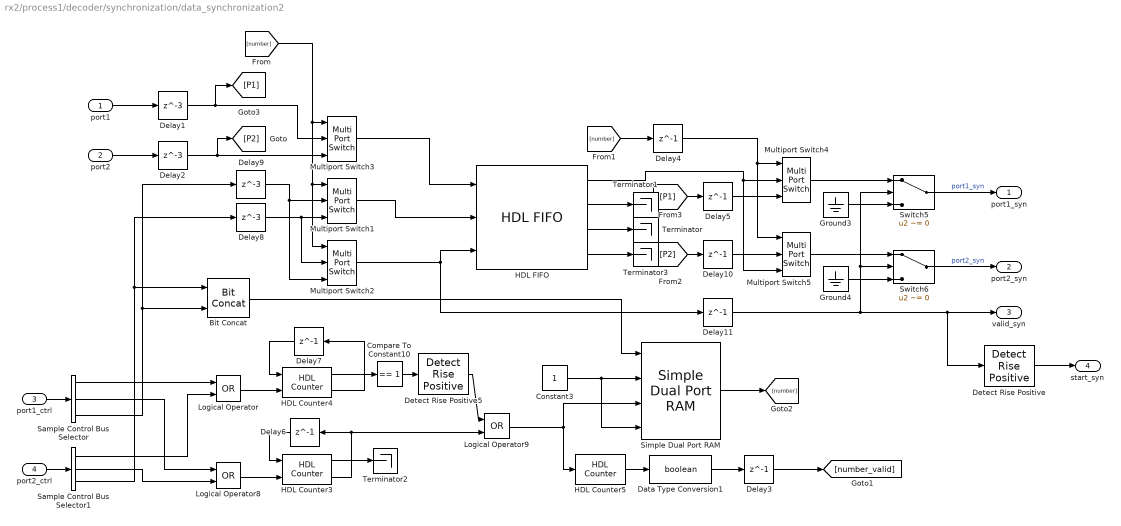
== system rx2/process1/decoder/synchronization/data_synchronization2 ==
  port1 : Inport
  port2 : Inport  Port=2
  port1_ctrl : Inport  Port=3  OutDataTypeStr=Bus: samplecontrol
  port2_ctrl : Inport  Port=4  OutDataTypeStr=Bus: samplecontrol
  Bit Concat : hdlsllib/Logic and Bit Operations/Bit Concat  numInputs=2
  Compare To Constant10 : hdlsllib/Logic and Bit Operations/Compare To Constant  relop===  const=1  OutDataTypeStr=boolean
  Constant3 : Constant  OutDataTypeStr=fixdt(0,2,0)
  Data Type Conversion1 : DataTypeConversion  OutDataTypeStr=boolean  SaturateOnIntegerOverflow=off  RndMeth=Floor
  Delay1 : Delay  DelayLength=3  InitialCondition=0  SampleTime=1
  Delay{3..7,10..11} (7 alike) : Delay  DelayLength=1  InitialCondition=0
  Delay2 : Delay  DelayLength=3  InitialCondition=0  SampleTime=1
  Delay8 : Delay  DelayLength=3  InitialCondition=0
  Delay9 : Delay  DelayLength=3  InitialCondition=0
  Detect Rise Positive : simulink/Logic and Bit Operations/Detect Rise Positive  vinit=0  OutDataTypeStr=boolean
  Detect Rise Positive5 : hdlsllib/Logic and Bit Operations/Detect Rise Positive  vinit=0  OutDataTypeStr=boolean
  Ground3 : Ground
  Ground4 : Ground
  HDL Counter3 : hdlsllib/Sources/HDL Counter  CountType=Count limited  CountInit=0  CountStep=1  CountMax=2  CountFromType=Initial value  CountFrom=0  CountResetPort=on  CountLoadPort=off  CountEnbPort=on  CountDirPort=off  CountHitOutputPort=on  CountDataType=Unsigned  CountWordLen=2  CountFracLen=0  CountSampTime=1
  HDL Counter4 : hdlsllib/Sources/HDL Counter  CountType=Count limited  CountInit=0  CountStep=1  CountMax=2  CountFromType=Initial value  CountFrom=0  CountResetPort=on  CountLoadPort=off  CountEnbPort=on  CountDirPort=off  CountHitOutputPort=on  CountDataType=Unsigned  CountWordLen=2  CountFracLen=0  CountSampTime=1
  HDL Counter5 : hdlsllib/Sources/HDL Counter  CountType=Count limited  CountInit=0  CountStep=1  CountMax=1  CountFromType=Initial value  CountFrom=0  CountResetPort=off  CountLoadPort=off  CountEnbPort=on  CountDirPort=off  CountHitOutputPort=off  CountDataType=Unsigned  CountWordLen=1  CountFracLen=0  CountSampTime=1
  HDL FIFO : hdlsllib/HDL RAMs/HDL FIFO  fifo_size=792  mode=Classic  ratio=1  push_msg=Warning  pop_msg=Ignore  show_empty=on  show_full=on  show_num=on  LabelModeActiveChoice_Mode=Classic  rst_port=off
  Logical Operator : Logic  Operator=OR  AllPortsSameDT=off  OutDataTypeStr=boolean
  Logical Operator8 : Logic  Operator=OR  AllPortsSameDT=off  OutDataTypeStr=boolean
  Logical Operator9 : Logic  Operator=OR  AllPortsSameDT=off  OutDataTypeStr=boolean
  Multiport Switch{1..5} (5 alike) : MultiPortSwitch  Inputs=2  DiagnosticForDefault=None  SaturateOnIntegerOverflow=off  InputSameDT=off
  Sample Control Bus Selector : whdlutilities/Sample Control Bus Selector  OutputSignals=start,end,valid
  Sample Control Bus Selector1 : whdlutilities/Sample Control Bus Selector  OutputSignals=start,end,valid
  Simple Dual Port RAM : hdlsllib/HDL RAMs/Simple Dual Port RAM  ram_size=2
  Switch5 : Switch  Criteria=u2 ~= 0  SaturateOnIntegerOverflow=off  InputSameDT=off
  Switch6 : Switch  Criteria=u2 ~= 0  SaturateOnIntegerOverflow=off  InputSameDT=off
  Terminator{,1..3} (4 alike) : Terminator
  port1_syn : Outport  VectorParamsAs1DForOutWhenUnconnected=off
  port2_syn : Outport  Port=2  VectorParamsAs1DForOutWhenUnconnected=off
  valid_syn : Outport  Port=3  OutDataTypeStr=boolean  VectorParamsAs1DForOutWhenUnconnected=off
  start_syn : Outport  Port=4  OutDataTypeStr=boolean  VectorParamsAs1DForOutWhenUnconnected=off
  wires:
  Detect Rise Positive/1 -> start_syn/1
  Delay11/1 -> valid_syn/1, Detect Rise Positive/1, Switch6/2, Switch5/2
  Multiport Switch5/1 -> Switch6/1
  Multiport Switch4/1 -> Switch5/1
  Ground3/1 -> Switch5/3
  Switch6/1 -> port2_syn/1  "port2_syn"
  Switch5/1 -> port1_syn/1  "port1_syn"
  Ground4/1 -> Switch6/3
  Delay5/1 -> Multiport Switch4/3
  Delay10/1 -> Multiport Switch5/2
  [P2] -> Delay10/1
  [P1] -> Delay5/1
  Delay1/1 -> Multiport Switch3/2, [P1]
  Delay4/1 -> Multiport Switch4/1, Multiport Switch5/1
  [number] -> Delay4/1
  HDL FIFO/4 -> Terminator3/1
  HDL FIFO/2 -> Terminator1/1
  Delay9/1 -> Multiport Switch1/2, Multiport Switch2/3
  Delay8/1 -> Multiport Switch1/3, Multiport Switch2/2
  Delay3/1 -> [number_valid]
  Delay2/1 -> Multiport Switch3/3, [P2]
  Sample Control Bus Selector1/3 -> Bit Concat/1, Delay8/1
  Sample Control Bus Selector/3 -> Bit Concat/2, Delay9/1
  [number] -> Multiport Switch3/1, Multiport Switch1/1, Multiport Switch2/1
  Multiport Switch2/1 -> Delay11/1, HDL FIFO/3
  Multiport Switch3/1 -> HDL FIFO/1
  HDL FIFO/3 -> Terminator/1
  HDL FIFO/1 -> Multiport Switch4/2, Multiport Switch5/3
  Multiport Switch1/1 -> HDL FIFO/2
  port2/1 -> Delay2/1
  port1/1 -> Delay1/1
  Simple Dual Port RAM/1 -> [number]
  Sample Control Bus Selector1/2 -> Logical Operator8/2
  Data Type Conversion1/1 -> Delay3/1
  Constant3/1 -> Simple Dual Port RAM/2, Simple Dual Port RAM/4
  Bit Concat/1 -> Simple Dual Port RAM/1
  Logical Operator9/1 -> Simple Dual Port RAM/3, HDL Counter5/1
  HDL Counter5/1 -> Data Type Conversion1/1
  HDL Counter4/1 -> Compare To Constant10/1
  Detect Rise Positive5/1 -> Logical Operator9/1
  Logical Operator/1 -> HDL Counter4/2
  Delay6/1 -> HDL Counter3/1
  HDL Counter3/1 -> Terminator2/1
  HDL Counter3/2 -> Delay6/1, Logical Operator9/2
  Logical Operator8/1 -> HDL Counter3/2
  Compare To Constant10/1 -> Detect Rise Positive5/1
  HDL Counter4/2 -> Delay7/1
  Delay7/1 -> HDL Counter4/1
  Sample Control Bus Selector/2 -> Logical Operator8/1
  Sample Control Bus Selector1/1 -> Logical Operator/2
  Sample Control Bus Selector/1 -> Logical Operator/1
  port2_ctrl/1 -> Sample Control Bus Selector1/1
  port1_ctrl/1 -> Sample Control Bus Selector/1

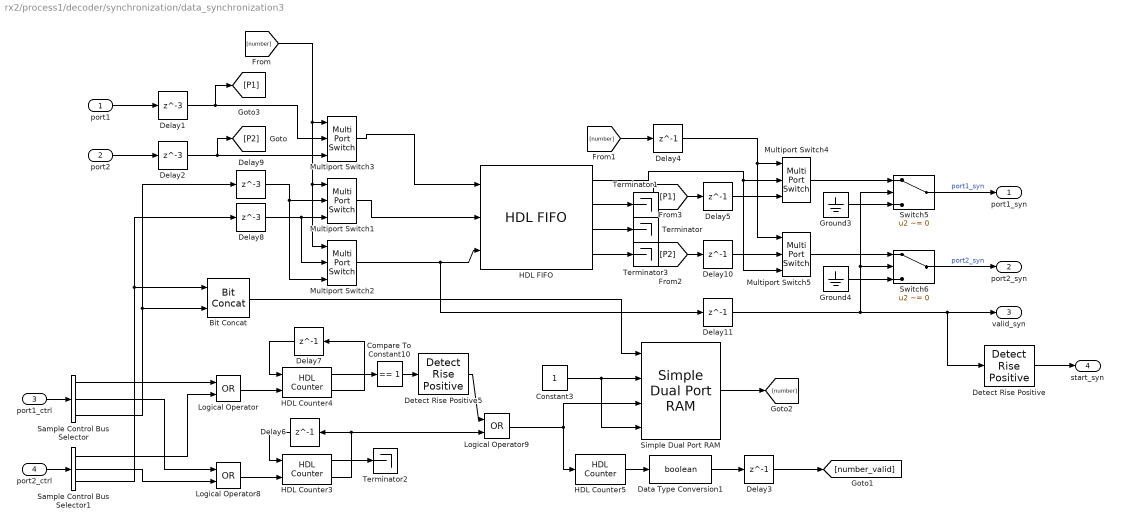
== system rx2/process1/decoder/synchronization/data_synchronization3 ==
  port1 : Inport
  port2 : Inport  Port=2
  port1_ctrl : Inport  Port=3  OutDataTypeStr=Bus: samplecontrol
  port2_ctrl : Inport  Port=4  OutDataTypeStr=Bus: samplecontrol
  Bit Concat : hdlsllib/Logic and Bit Operations/Bit Concat  numInputs=2
  Compare To Constant10 : hdlsllib/Logic and Bit Operations/Compare To Constant  relop===  const=1  OutDataTypeStr=boolean
  Constant3 : Constant  OutDataTypeStr=fixdt(0,2,0)
  Data Type Conversion1 : DataTypeConversion  OutDataTypeStr=boolean  SaturateOnIntegerOverflow=off  RndMeth=Floor
  Delay1 : Delay  DelayLength=3  InitialCondition=0  SampleTime=1
  Delay{3..7,10..11} (7 alike) : Delay  DelayLength=1  InitialCondition=0
  Delay2 : Delay  DelayLength=3  InitialCondition=0  SampleTime=1
  Delay8 : Delay  DelayLength=3  InitialCondition=0
  Delay9 : Delay  DelayLength=3  InitialCondition=0
  Detect Rise Positive : simulink/Logic and Bit Operations/Detect Rise Positive  vinit=0  OutDataTypeStr=boolean
  Detect Rise Positive5 : hdlsllib/Logic and Bit Operations/Detect Rise Positive  vinit=0  OutDataTypeStr=boolean
  Ground3 : Ground
  Ground4 : Ground
  HDL Counter3 : hdlsllib/Sources/HDL Counter  CountType=Count limited  CountInit=0  CountStep=1  CountMax=2  CountFromType=Initial value  CountFrom=0  CountResetPort=on  CountLoadPort=off  CountEnbPort=on  CountDirPort=off  CountHitOutputPort=on  CountDataType=Unsigned  CountWordLen=2  CountFracLen=0  CountSampTime=1
  HDL Counter4 : hdlsllib/Sources/HDL Counter  CountType=Count limited  CountInit=0  CountStep=1  CountMax=2  CountFromType=Initial value  CountFrom=0  CountResetPort=on  CountLoadPort=off  CountEnbPort=on  CountDirPort=off  CountHitOutputPort=on  CountDataType=Unsigned  CountWordLen=2  CountFracLen=0  CountSampTime=1
  HDL Counter5 : hdlsllib/Sources/HDL Counter  CountType=Count limited  CountInit=0  CountStep=1  CountMax=1  CountFromType=Initial value  CountFrom=0  CountResetPort=off  CountLoadPort=off  CountEnbPort=on  CountDirPort=off  CountHitOutputPort=off  CountDataType=Unsigned  CountWordLen=1  CountFracLen=0  CountSampTime=1
  HDL FIFO : hdlsllib/HDL RAMs/HDL FIFO  fifo_size=792  mode=Classic  ratio=1  push_msg=Warning  pop_msg=Ignore  show_empty=on  show_full=on  show_num=on  LabelModeActiveChoice_Mode=Classic  rst_port=off
  Logical Operator : Logic  Operator=OR  AllPortsSameDT=off  OutDataTypeStr=boolean
  Logical Operator8 : Logic  Operator=OR  AllPortsSameDT=off  OutDataTypeStr=boolean
  Logical Operator9 : Logic  Operator=OR  AllPortsSameDT=off  OutDataTypeStr=boolean
  Multiport Switch{1..5} (5 alike) : MultiPortSwitch  Inputs=2  DiagnosticForDefault=None  SaturateOnIntegerOverflow=off  InputSameDT=off
  Sample Control Bus Selector : whdlutilities/Sample Control Bus Selector  OutputSignals=start,end,valid
  Sample Control Bus Selector1 : whdlutilities/Sample Control Bus Selector  OutputSignals=start,end,valid
  Simple Dual Port RAM : hdlsllib/HDL RAMs/Simple Dual Port RAM  ram_size=2
  Switch5 : Switch  Criteria=u2 ~= 0  SaturateOnIntegerOverflow=off  InputSameDT=off
  Switch6 : Switch  Criteria=u2 ~= 0  SaturateOnIntegerOverflow=off  InputSameDT=off
  Terminator{,1..3} (4 alike) : Terminator
  port1_syn : Outport  VectorParamsAs1DForOutWhenUnconnected=off
  port2_syn : Outport  Port=2  VectorParamsAs1DForOutWhenUnconnected=off
  valid_syn : Outport  Port=3  OutDataTypeStr=boolean  VectorParamsAs1DForOutWhenUnconnected=off
  start_syn : Outport  Port=4  OutDataTypeStr=boolean  VectorParamsAs1DForOutWhenUnconnected=off
  wires:
  Detect Rise Positive/1 -> start_syn/1
  Delay11/1 -> valid_syn/1, Detect Rise Positive/1, Switch6/2, Switch5/2
  Multiport Switch5/1 -> Switch6/1
  Multiport Switch4/1 -> Switch5/1
  Ground3/1 -> Switch5/3
  Switch6/1 -> port2_syn/1  "port2_syn"
  Switch5/1 -> port1_syn/1  "port1_syn"
  Ground4/1 -> Switch6/3
  Delay5/1 -> Multiport Switch4/3
  Delay10/1 -> Multiport Switch5/2
  [P2] -> Delay10/1
  [P1] -> Delay5/1
  Delay1/1 -> Multiport Switch3/2, [P1]
  Delay4/1 -> Multiport Switch4/1, Multiport Switch5/1
  [number] -> Delay4/1
  HDL FIFO/4 -> Terminator3/1
  HDL FIFO/2 -> Terminator1/1
  Delay9/1 -> Multiport Switch1/2, Multiport Switch2/3
  Delay8/1 -> Multiport Switch1/3, Multiport Switch2/2
  Delay3/1 -> [number_valid]
  Delay2/1 -> Multiport Switch3/3, [P2]
  Sample Control Bus Selector1/3 -> Bit Concat/1, Delay8/1
  Sample Control Bus Selector/3 -> Bit Concat/2, Delay9/1
  [number] -> Multiport Switch3/1, Multiport Switch1/1, Multiport Switch2/1
  Multiport Switch2/1 -> Delay11/1, HDL FIFO/3
  Multiport Switch3/1 -> HDL FIFO/1
  HDL FIFO/3 -> Terminator/1
  HDL FIFO/1 -> Multiport Switch4/2, Multiport Switch5/3
  Multiport Switch1/1 -> HDL FIFO/2
  port2/1 -> Delay2/1
  port1/1 -> Delay1/1
  Simple Dual Port RAM/1 -> [number]
  Sample Control Bus Selector1/2 -> Logical Operator8/2
  Data Type Conversion1/1 -> Delay3/1
  Constant3/1 -> Simple Dual Port RAM/2, Simple Dual Port RAM/4
  Bit Concat/1 -> Simple Dual Port RAM/1
  Logical Operator9/1 -> Simple Dual Port RAM/3, HDL Counter5/1
  HDL Counter5/1 -> Data Type Conversion1/1
  HDL Counter4/1 -> Compare To Constant10/1
  Detect Rise Positive5/1 -> Logical Operator9/1
  Logical Operator/1 -> HDL Counter4/2
  Delay6/1 -> HDL Counter3/1
  HDL Counter3/1 -> Terminator2/1
  HDL Counter3/2 -> Delay6/1, Logical Operator9/2
  Logical Operator8/1 -> HDL Counter3/2
  Compare To Constant10/1 -> Detect Rise Positive5/1
  HDL Counter4/2 -> Delay7/1
  Delay7/1 -> HDL Counter4/1
  Sample Control Bus Selector/2 -> Logical Operator8/1
  Sample Control Bus Selector1/1 -> Logical Operator/2
  Sample Control Bus Selector/1 -> Logical Operator/1
  port2_ctrl/1 -> Sample Control Bus Selector1/1
  port1_ctrl/1 -> Sample Control Bus Selector/1
